simulink model "leg_contral_from_joy"  (R2024a)
settings: Solver=FixedStepDiscrete  StartTime=0.0  StopTime=inf  FixedStep=0.01  RelTol=1e-3  EnableMultiTasking=on
InitFcn:
  | run('robota_init.m')
values from neighbouring files (symbols this model uses):
  foot_step_x = single([0.647962241881123,0.669281948440417,0.689047458853030,0.707336632089232,0.724214871275340,0.739734081466605,0.753932398834638,0.766834545548556,0.778452679930586,0.788787625824203,0.797830378556315,0.805563797434742,0.811964406427908,0.817004235554845,0.820652645599333,0.822878088081130,0.823649760998204,0.822939128724922,0.820721281639968,0.816976117592065,0.811689333218330,0.804853218436 ...(+3308 chars)    [robota_init.m]
  foot_step_y = single([0.00431677655718721,0.0162618273816606,0.0344599539851875,0.0576998848000865,0.0849190036162384,0.115189239656799,0.147704049746776,0.181766425758056,0.216777863221598,0.252228229678260,0.287686473989677,0.322792120445942,0.357247494083859,0.390810626164481,0.423288791248474,0.454532629749211,0.484430812233581,0.512905204076631,0.539906491355785,0.565410231091200,0.589413291098898,0.611930 ...(+3410 chars)    [robota_init.m]
  height_plane = 0.025    [robota_init.m]
undefined symbols (not defined in the file or in its folder): axes, axes_SL_Info, buttons, buttons_SL_Info, foot_z, header, lb_alfa, lb_beta, lb_gamma, lf_alfa, lf_beta, lf_gamma, plane_x, plane_y, rb_alfa, rb_beta, rb_gamma, rf_alfa, rf_beta, rf_gamma, x, X, y, Y, z, Z
libraries: sm_lib x84, nesl_utility x21, hdlsllib x20, ros2lib x10, instrumentseriallib x2
(part 1 of 3)
settings Model: SimulationMode=external  Creator=The MathWorks, Inc.  LastModifiedBy=yang
settings SolverCC: AlgebraicLoopSolver=TrustRegion  PositivePriorityOrder=on
settings DataIOCC: LimitDataPoints=on  SaveFormat=Array  ReturnWorkspaceOutputs=off
settings OptimizationCC: ZeroExternalMemoryAtStartup=off  ZeroInternalMemoryAtStartup=off  LifeSpan=1  MaxStackSize=64
settings DebuggingCC: SolverPrmCheckMsg=warning  UnconnectedInputMsg=warning  UnconnectedOutputMsg=warning  UnconnectedLineMsg=warning  SFUnexpectedBacktrackingDiag=warning  SFNoUnconditionalDefaultTransitionDiag=warning  SFExecutionAtInitializationDiag=none  ArithmeticOperatorsInVariantConditions=warning
settings HardwareCC: ProdBitPerLong=64  ProdHWDeviceType=AMD->x86-64 (Linux 64)  TargetHWDeviceType=Generic->Unspecified (assume 32-bit Generic)
settings ModelReferenceCC: EnableRefExpFcnMdlSchedulingChecks=on  ModelReferenceNumInstancesAllowed=Single  PropagateSignalLabelsOutOfModel=off
settings SFSimCC: SimUseLocalCustomCode=off  SimTargetLang=C++
settings RTWCC: Description=Embedded Coder  SystemTargetFile=ert.tlc  HardwareBoard=Robot Operating System 2 (ROS 2)  TLCOptions="-aInlineSetEventsForThisBaseRateFcn=TLC_FALSE -aSuppressMultiTaskScheduler=TLC_FALSE   -aRateBasedStepFcn=0"  TemplateMakefile=ert_default_tmf  RTWUseLocalCustomCode=off  Toolchain=Colcon Tools  TargetLang=C++  GPUComputeCapability=3.5
settings CodeAppCC: StateflowObjectComments=on
settings ERTTargetCC: MultiwordLength=2048  ERTCustomFileBanners=off  CodeInterfacePackaging=C++ class  SupportContinuousTime=on  SupportNonInlinedSFcns=on  RemoveResetFunc=off  SupportVariableSizeSignals=on  ModelStepFunctionPrototypeControlCompliant=off  RootIOFormat=Structure reference  ConvertIfToSwitch=off  SuppressUnreachableDefaultCases=off
settings ConfigComp: CovMetricSettings=dw  CovSaveCumulativeToWorkspaceVar=on  CovSaveSingleToWorkspaceVar=on  CovExternalEMLEnable=off  CovSFcnEnable=off

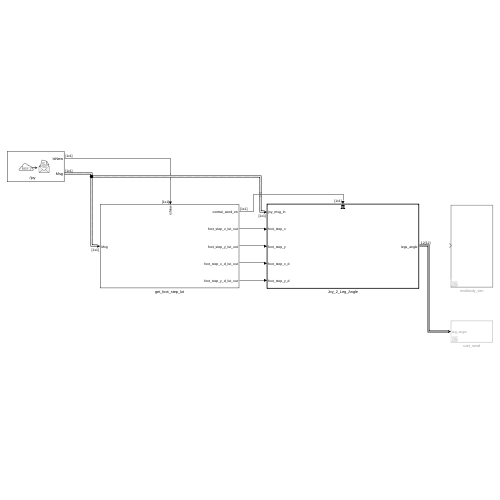
[thumbnail: Simulink's stored preview of the top-level diagram]
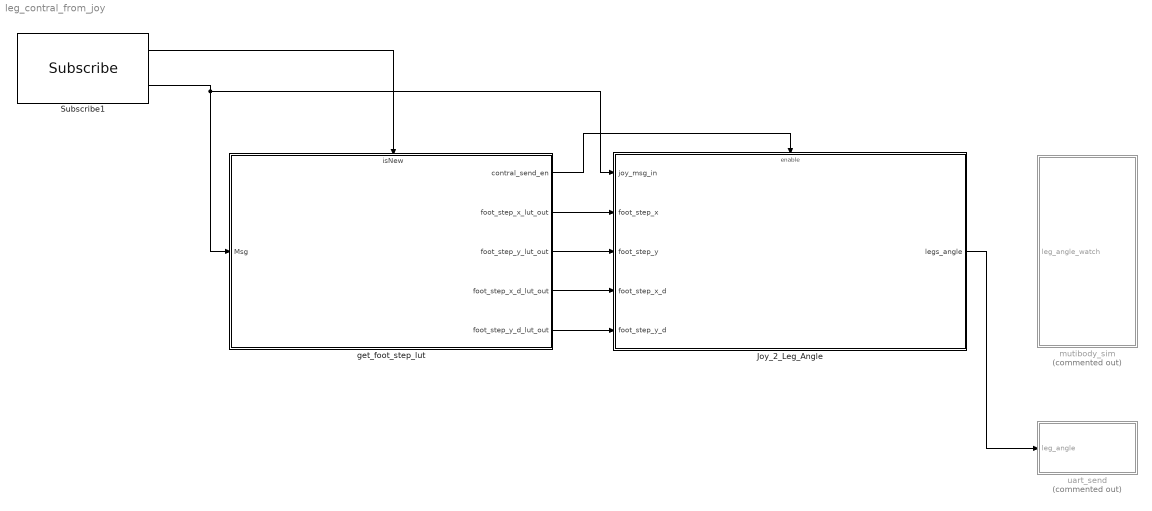
== system leg_contral_from_joy ==
  Joy_2_Leg_Angle : Subsystem
  Subscribe1 : ros2lib/Subscribe  topicSource=Select from ROS network  topic=/joy  messageType=sensor_msgs/Joy  sampleTime=0.01  QOSHistory=Keep last  QOSDepth=1  QOSReliability=Reliable  QOSDurability=Volatile  QOSDeadline=Inf  QOSLifespan=Inf  QOSLiveliness=Automatic  QOSLeaseDuration=Inf  QOSAvoidROSNamespaceConventions=off
  get_foot_step_lut : Subsystem
      settings: PortSchema="{\"entries\":[{\"content\":{\"sides\":[{\"content\":{\"connectorIds\":[\"In1\"]},\"type\":\"ConnectorPlacement.EquallySpacedRectSide\",\"uuid\":\"62496544-86df-4f58-acc1-b6358197f44c\"},{\"content\":{\"connectorIds\":[\"Out1\",\"Out2\",\"Out3\",\"Out4\",\"Out5\"],\"side\":\"RIGHT\"},\"type\":\"ConnectorPlacement.EquallySpacedRectSide\",\"uuid\":\"00f5c7b2-a8b0-46a5-a80f-764e0da961ac\"},{\"content\":{\"connectorIds\":[\"In2\"],\"side\":\"TOP\"},\"type\":\"ConnectorPlacement.EquallySpacedRectSide\",\"uuid\":\"1933786d-7f7d-47a2-bd92-b828693c7f9d\"}]},\"type\":\"ConnectorPlacement.EquallySpacedConnector\",\"uuid\":\"7dc846c5-42fe-4877-a1f3-97792b9a7f59\"}],\"packageUris\":[\"http://schema.mathworks.com/mf0/Connector/R2020b\"],\"version\":\"1.0\"}"
  mutibody_sim : Subsystem  Commented=on  TreatAsAtomicUnit=on
  uart_send : Subsystem  Commented=on
  wires:
  Subscribe1/2 -> Joy_2_Leg_Angle/1(joy_msg_in), get_foot_step_lut/1(Msg)
  Subscribe1/1 -> get_foot_step_lut/2(isNew)
  get_foot_step_lut/1(contral_send_en) -> Joy_2_Leg_Angle/Enable
  get_foot_step_lut/2(foot_step_x_lut_out) -> Joy_2_Leg_Angle/2(foot_step_x)
  get_foot_step_lut/3(foot_step_y_lut_out) -> Joy_2_Leg_Angle/3(foot_step_y)
  get_foot_step_lut/4(foot_step_x_d_lut_out) -> Joy_2_Leg_Angle/4(foot_step_x_d)
  get_foot_step_lut/5(foot_step_y_d_lut_out) -> Joy_2_Leg_Angle/5(foot_step_y_d)
  Joy_2_Leg_Angle/1(legs_angle) -> uart_send/1(leg_angle)

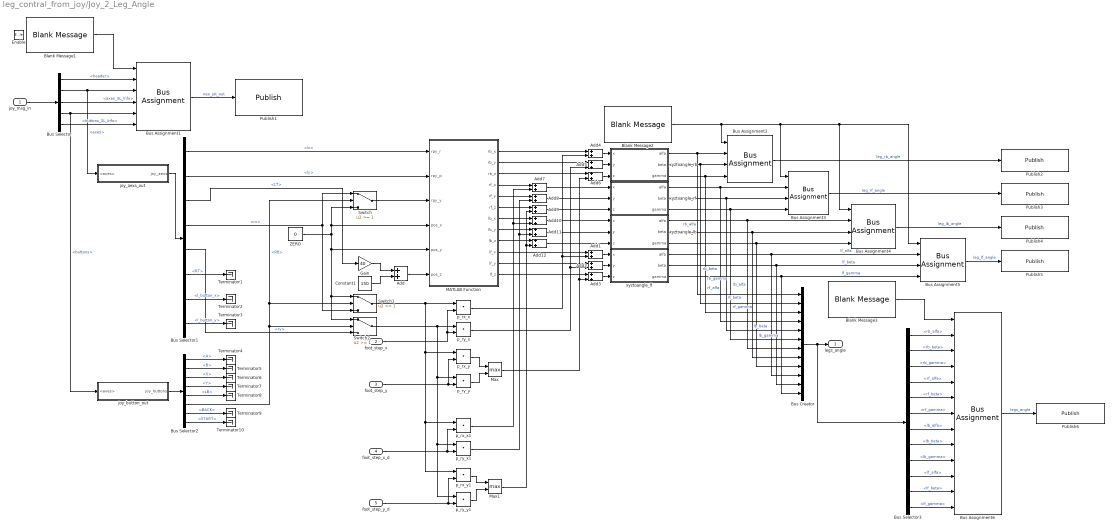
== system leg_contral_from_joy/Joy_2_Leg_Angle ==
  joy_msg_in : Inport
  foot_step_x : Inport  Port=2
  foot_step_y : Inport  Port=3
  foot_step_x_d : Inport  Port=4
  foot_step_y_d : Inport  Port=5
  Enable : EnablePort
  Add{,1..12} (13 alike) : Sum
  Blank Message1 : ros2lib/Blank Message  messageClass=Message  entityType=sensor_msgs/Joy  messageType=sensor_msgs/Joy  SampleTime=0.01
  Blank Message2 : ros2lib/Blank Message  messageClass=Message  entityType=geometry_msgs/Vector3  messageType=geometry_msgs/Vector3  SampleTime=0.01
  Blank Message3 : ros2lib/Blank Message  messageClass=Message  entityType=robota_leg_pos/LegPos  messageType=robota_leg_pos/LegPos  SampleTime=0.01
  Bus Assignment1 : BusAssignment  AssignedSignals=header,axes,axes_SL_Info,buttons,buttons_SL_Info
  Bus Assignment{2..5} (4 alike) : BusAssignment  AssignedSignals=x,y,z
  Bus Assignment6 : BusAssignment  AssignedSignals=rb_alfa,rb_beta,rb_gamma,rf_alfa,rf_beta,rf_gamma,lb_alfa,lb_beta,lb_gamma,lf_alfa,lf_beta,lf_gamma
  Bus Creator : BusCreator  Inputs=12
  Bus Selector : BusSelector  DialogController=Simulink.DDGSource_BusSelector  OutputSignals=header,axes,axes_SL_Info,buttons,buttons_SL_Info
  Bus Selector1 : BusSelector  OutputSignals=lx,ly,LT,rx,ry,RT,l_button_x,l_button_y
  Bus Selector2 : BusSelector  OutputSignals=A,B,X,Y,LB,RB,BACK,START
  Bus Selector3 : BusSelector  OutputSignals=rb_alfa,rb_beta,rb_gamma,rf_alfa,rf_beta,rf_gamma,lb_alfa,lb_beta,lb_gamma,lf_alfa,lf_beta,lf_gamma
  Constant1 : Constant  Value=150  SampleTime=0.01
  Gain : Gain  Gain=40
  MATLAB Function : MATLAB Function  TreatAsAtomicUnit=on
  Max : MinMax  Function=max  Inputs=2
  Max1 : MinMax  Function=max  Inputs=2
  Publish1 : ros2lib/Publish  topicSource=Specify your own  topic=/joy_neo  messageType=sensor_msgs/Joy  QOSHistory=Keep last  QOSDepth=10  QOSReliability=Reliable  QOSDurability=Volatile  QOSDeadline=Inf  QOSLifespan=Inf  QOSLiveliness=Automatic  QOSLeaseDuration=Inf  QOSAvoidROSNamespaceConventions=off
  Publish2 : ros2lib/Publish  topicSource=Specify your own  topic=/leg_rb_angle  messageType=geometry_msgs/Vector3  QOSHistory=Keep last  QOSDepth=10  QOSReliability=Reliable  QOSDurability=Volatile  QOSDeadline=Inf  QOSLifespan=Inf  QOSLiveliness=Automatic  QOSLeaseDuration=Inf  QOSAvoidROSNamespaceConventions=off
  Publish3 : ros2lib/Publish  topicSource=Specify your own  topic=/leg_rf_angle  messageType=geometry_msgs/Vector3  QOSHistory=Keep last  QOSDepth=10  QOSReliability=Reliable  QOSDurability=Volatile  QOSDeadline=Inf  QOSLifespan=Inf  QOSLiveliness=Automatic  QOSLeaseDuration=Inf  QOSAvoidROSNamespaceConventions=off
  Publish4 : ros2lib/Publish  topicSource=Specify your own  topic=/leg_lb_angle  messageType=geometry_msgs/Vector3  QOSHistory=Keep last  QOSDepth=10  QOSReliability=Reliable  QOSDurability=Volatile  QOSDeadline=Inf  QOSLifespan=Inf  QOSLiveliness=Automatic  QOSLeaseDuration=Inf  QOSAvoidROSNamespaceConventions=off
  Publish5 : ros2lib/Publish  topicSource=Specify your own  topic=/leg_lf_angle  messageType=geometry_msgs/Vector3  QOSHistory=Keep last  QOSDepth=10  QOSReliability=Reliable  QOSDurability=Volatile  QOSDeadline=Inf  QOSLifespan=Inf  QOSLiveliness=Automatic  QOSLeaseDuration=Inf  QOSAvoidROSNamespaceConventions=off
  Publish6 : ros2lib/Publish  topicSource=Specify your own  topic=/legs_angle  messageType=robota_leg_pos/LegPos  QOSHistory=Keep last  QOSDepth=10  QOSReliability=Reliable  QOSDurability=Volatile  QOSDeadline=Inf  QOSLifespan=Inf  QOSLiveliness=Automatic  QOSLeaseDuration=Inf  QOSAvoidROSNamespaceConventions=off
  Switch : Switch  Threshold=1  SaturateOnIntegerOverflow=off  InputSameDT=off
  Switch1 : Switch  Threshold=1  SaturateOnIntegerOverflow=off  InputSameDT=off
  Switch2 : Switch  Threshold=1  SaturateOnIntegerOverflow=off  InputSameDT=off
  Terminator{1..10} (10 alike) : Terminator
  ZERO : Constant  Value=0  SampleTime=0.01
  joy_aexs_out : Subsystem
  joy_button_out : Subsystem
  p_rx_x : DotProduct  OutDataTypeStr=single
  p_rx_x1 : DotProduct  OutDataTypeStr=Inherit: Inherit via internal rule
  p_rx_y : DotProduct  OutDataTypeStr=Inherit: Inherit via internal rule
  p_rx_y1 : DotProduct  OutDataTypeStr=Inherit: Inherit via internal rule
  p_ry_x : DotProduct  OutDataTypeStr=Inherit: Inherit via internal rule
  p_ry_x1 : DotProduct  OutDataTypeStr=Inherit: Inherit via internal rule
  p_ry_y : DotProduct  OutDataTypeStr=Inherit: Inherit via internal rule
  p_ry_y1 : DotProduct  OutDataTypeStr=Inherit: Inherit via internal rule
  xyztoangle_lb : MATLAB Function  TreatAsAtomicUnit=on
  xyztoangle_lf : MATLAB Function  TreatAsAtomicUnit=on
  xyztoangle_rb : MATLAB Function  TreatAsAtomicUnit=on
  xyztoangle_rf : MATLAB Function  TreatAsAtomicUnit=on
  legs_angle : Outport
  wires:
  joy_msg_in/1 -> Bus Selector/1
  Bus Selector/2 -> Bus Assignment1/3, joy_aexs_out/1(<axes>)  "<axes>"
  Blank Message1/1 -> Bus Assignment1/1
  Bus Assignment1/1 -> Publish1/1  "neo_jot_out"
  Bus Selector/4 -> joy_button_out/1(<axes>), Bus Assignment1/5  "<buttons>"
  Bus Selector/1 -> Bus Assignment1/2  "<header>"
  Bus Selector/3 -> Bus Assignment1/4  "<axes_SL_Info>"
  Bus Selector/5 -> Bus Assignment1/6  "<buttons_SL_Info>"
  MATLAB Function/1(rb_x) -> Add4/1
  MATLAB Function/2(rb_y) -> Add5/1
  MATLAB Function/3(rb_z) -> Add6/1
  MATLAB Function/4(rf_x) -> Add7/1
  MATLAB Function/5(rf_y) -> Add8/1
  MATLAB Function/6(rf_z) -> Add9/1
  MATLAB Function/7(lb_x) -> Add10/1
  MATLAB Function/8(lb_y) -> Add11/1
  MATLAB Function/9(lb_z) -> Add12/1
  MATLAB Function/10(lf_x) -> Add1/1
  MATLAB Function/11(lf_y) -> Add2/1
  MATLAB Function/12(lf_z) -> Add3/1
  joy_aexs_out/1(joy_aexs) -> Bus Selector1/1
  Bus Selector1/1 -> MATLAB Function/1(rpy_r)  "<lx>"
  Bus Selector1/2 -> MATLAB Function/2(rpy_p)  "<ly>"
  Bus Selector1/3 -> Gain/1  "<LT>"
  Bus Selector1/6 -> Terminator1/1  "<RT>"
  Bus Selector1/8 -> Terminator3/1  "<l_button_y>"
  ZERO/1 -> MATLAB Function/5(pos_y), Switch2/1, Switch1/1, MATLAB Function/4(pos_x), Switch/3
  Add/1 -> MATLAB Function/6(pos_z)
  Blank Message2/1 -> Bus Assignment5/1, Bus Assignment4/1, Bus Assignment3/1, Bus Assignment2/1
  xyztoangle_rb/1(alfa) -> Bus Creator/1, Bus Assignment2/2  "rb_alfa"
  xyztoangle_rb/2(beta) -> Bus Creator/2, Bus Assignment2/3  "rb_beta"
  xyztoangle_rb/3(gamma) -> Bus Creator/3, Bus Assignment2/4  "rb_gamma"
  Bus Assignment2/1 -> Publish2/1  "leg_rb_angle"
  Bus Assignment3/1 -> Publish3/1  "leg_rf_angle"
  xyztoangle_rf/1(alfa) -> Bus Creator/4, Bus Assignment3/2  "rf_alfa"
  xyztoangle_rf/2(beta) -> Bus Creator/5, Bus Assignment3/3  "rf_beta"
  xyztoangle_rf/3(gamma) -> Bus Creator/6, Bus Assignment3/4  "rf_gamma"
  Bus Assignment5/1 -> Publish5/1  "leg_lf_angle"
  Bus Assignment4/1 -> Publish4/1  "leg_lb_angle"
  xyztoangle_lb/1(alfa) -> Bus Creator/7, Bus Assignment4/2  "lb_alfa"
  xyztoangle_lb/2(beta) -> Bus Creator/8, Bus Assignment4/3  "lb_beta"
  xyztoangle_lb/3(gamma) -> Bus Creator/9, Bus Assignment4/4  "lb_gamma"
  xyztoangle_lf/1(alfa) -> Bus Creator/10, Bus Assignment5/2  "lf_alfa"
  xyztoangle_lf/2(beta) -> Bus Creator/11, Bus Assignment5/3  "lf_beta"
  xyztoangle_lf/3(gamma) -> Bus Creator/12, Bus Assignment5/4  "lf_gamma"
  joy_button_out/1(joy_buttons) -> Bus Selector2/1
  Bus Selector2/1 -> Terminator4/1  "<A>"
  Bus Selector2/2 -> Terminator5/1  "<B>"
  Bus Selector2/3 -> Terminator6/1  "<X>"
  Bus Selector2/4 -> Terminator7/1  "<Y>"
  Bus Selector2/5 -> Terminator8/1  "<LB>"
  Bus Selector2/6 -> Switch1/2, Switch/2, Switch2/2  "<RB>"
  Bus Selector2/7 -> Terminator9/1  "<BACK>"
  Bus Selector2/8 -> Terminator10/1  "<START>"
  Switch/1 -> MATLAB Function/3(rpy_y)
  Constant1/1 -> Add/2
  Gain/1 -> Add/1
  Add1/1 -> xyztoangle_lf/1(x)
  Add2/1 -> xyztoangle_lf/2(y)
  Add3/1 -> xyztoangle_lf/3(z)
  foot_step_y/1 -> p_rx_y/2, p_ry_y/2
  p_rx_y/1 -> Max/1
  foot_step_x/1 -> p_rx_x/2, p_ry_x/2
  p_rx_x/1 -> Add4/2, Add1/2
  Max/1 -> Add6/2, Add3/2
  p_ry_y/1 -> Max/2
  p_ry_x/1 -> Add5/2, Add2/2
  Add4/1 -> xyztoangle_rb/1(x)
  Add5/1 -> xyztoangle_rb/2(y)
  Add6/1 -> xyztoangle_rb/3(z)
  foot_step_x_d/1 -> p_rx_x1/2, p_ry_x1/2
  foot_step_y_d/1 -> p_rx_y1/2, p_ry_y1/2
  Switch2/1 -> p_ry_x/1, p_ry_x1/1, p_ry_y1/1, p_ry_y/1
  Switch1/1 -> p_rx_y/1, p_rx_y1/1, p_rx_x1/1, p_rx_x/1
  p_rx_y1/1 -> Max1/1
  p_ry_y1/1 -> Max1/2
  Add7/1 -> xyztoangle_rf/1(x)
  Add8/1 -> xyztoangle_rf/2(y)
  Add9/1 -> xyztoangle_rf/3(z)
  Add10/1 -> xyztoangle_lb/1(x)
  Add11/1 -> xyztoangle_lb/2(y)
  Add12/1 -> xyztoangle_lb/3(z)
  p_rx_x1/1 -> Add10/2, Add7/2
  p_ry_x1/1 -> Add8/2, Add11/2
  Max1/1 -> Add9/2, Add12/2
  Bus Selector1/7 -> Terminator2/1  "<l_button_x>"
  Bus Selector1/4 -> Switch/1, Switch1/3  "<rx>"
  Bus Selector1/5 -> Switch2/3  "<ry>"
  Bus Creator/1 -> Bus Selector3/1, legs_angle/1
  Blank Message3/1 -> Bus Assignment6/1
  Bus Assignment6/1 -> Publish6/1  "legs_angle"
  Bus Selector3/1 -> Bus Assignment6/2  "<rb_alfa>"
  Bus Selector3/2 -> Bus Assignment6/3  "<rb_beta>"
  Bus Selector3/3 -> Bus Assignment6/4  "<rb_gamma>"
  Bus Selector3/4 -> Bus Assignment6/5  "<rf_alfa>"
  Bus Selector3/5 -> Bus Assignment6/6  "<rf_beta>"
  Bus Selector3/6 -> Bus Assignment6/7  "<rf_gamma>"
  Bus Selector3/7 -> Bus Assignment6/8  "<lb_alfa>"
  Bus Selector3/8 -> Bus Assignment6/9  "<lb_beta>"
  Bus Selector3/9 -> Bus Assignment6/10  "<lb_gamma>"
  Bus Selector3/10 -> Bus Assignment6/11  "<lf_alfa>"
  Bus Selector3/11 -> Bus Assignment6/12  "<lf_beta>"
  Bus Selector3/12 -> Bus Assignment6/13  "<lf_gamma>"

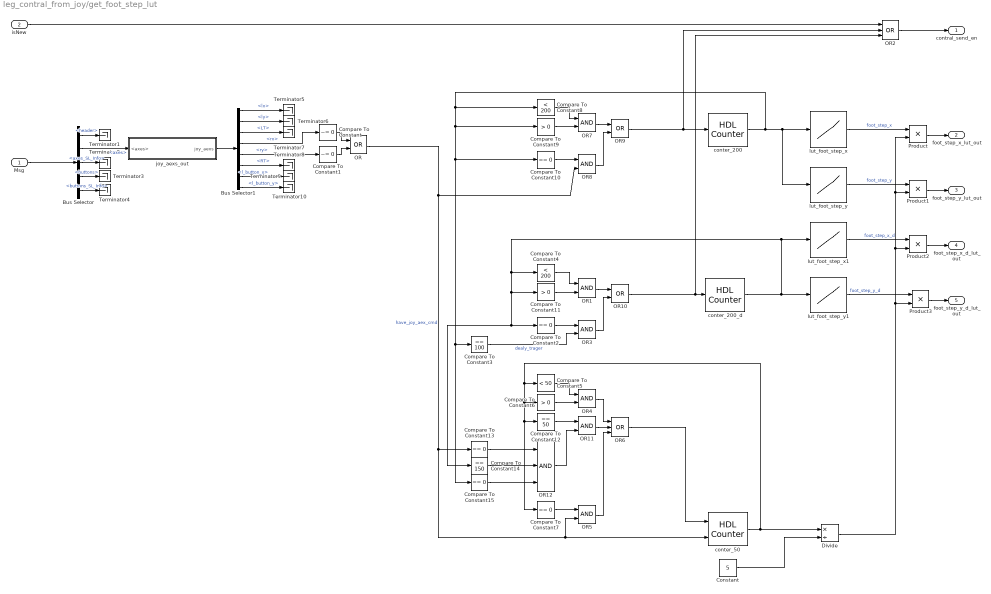
== system leg_contral_from_joy/get_foot_step_lut ==
  Msg : Inport
  isNew : Inport  Port=2
  Bus Selector : BusSelector  DialogController=Simulink.DDGSource_BusSelector  OutputSignals=header,axes,axes_SL_Info,buttons,buttons_SL_Info
  Bus Selector1 : BusSelector  OutputSignals=lx,ly,LT,rx,ry,RT,l_button_x,l_button_y
  Compare To Constant : hdlsllib/Logic and Bit Operations/Compare To Constant  relop=~=  const=0  OutDataTypeStr=boolean
  Compare To Constant1 : hdlsllib/Logic and Bit Operations/Compare To Constant  relop=~=  const=0  OutDataTypeStr=boolean
  Compare To Constant{2,7,10,13,15} (5 alike) : hdlsllib/Logic and Bit Operations/Compare To Constant  relop===  const=0  OutDataTypeStr=boolean
  Compare To Constant11 : hdlsllib/Logic and Bit Operations/Compare To Constant  relop=>  const=0  OutDataTypeStr=boolean
  Compare To Constant12 : hdlsllib/Logic and Bit Operations/Compare To Constant  relop===  const=50  OutDataTypeStr=boolean
  Compare To Constant14 : hdlsllib/Logic and Bit Operations/Compare To Constant  relop===  const=150  OutDataTypeStr=boolean
  Compare To Constant3 : hdlsllib/Logic and Bit Operations/Compare To Constant  relop===  const=100  OutDataTypeStr=boolean
  Compare To Constant4 : hdlsllib/Logic and Bit Operations/Compare To Constant  relop=<  const=200  OutDataTypeStr=boolean
  Compare To Constant5 : hdlsllib/Logic and Bit Operations/Compare To Constant  relop=<  const=50  OutDataTypeStr=boolean
  Compare To Constant6 : hdlsllib/Logic and Bit Operations/Compare To Constant  relop=>  const=0  OutDataTypeStr=boolean
  Compare To Constant8 : hdlsllib/Logic and Bit Operations/Compare To Constant  relop=<  const=200  OutDataTypeStr=boolean
  Compare To Constant9 : hdlsllib/Logic and Bit Operations/Compare To Constant  relop=>  const=0  OutDataTypeStr=boolean
  Constant : Constant  Value=5  SampleTime=0.01
  Divide : Product  Inputs=*/
  OR : Logic  Operator=OR  AllPortsSameDT=off  OutDataTypeStr=boolean
  OR{1,3..5,7..8,11} (7 alike) : Logic  AllPortsSameDT=off  OutDataTypeStr=boolean
  OR10 : Logic  Operator=OR  AllPortsSameDT=off  OutDataTypeStr=boolean
  OR12 : Logic  Inputs=3  AllPortsSameDT=off  OutDataTypeStr=boolean
  OR2 : Logic  Operator=OR  Inputs=3  AllPortsSameDT=off  OutDataTypeStr=boolean
  OR6 : Logic  Operator=OR  Inputs=3  AllPortsSameDT=off  OutDataTypeStr=boolean
  OR9 : Logic  Operator=OR  AllPortsSameDT=off  OutDataTypeStr=boolean
  Product{,1..3} (4 alike) : Product  OutDataTypeStr=single
  Terminator{1..10} (10 alike) : Terminator
  conter_200 : hdlsllib/Sources/HDL Counter  CountType=Count limited  CountInit=0  CountStep=1  CountMax=199  CountFromType=Initial value  CountFrom=0  CountResetPort=off  CountLoadPort=off  CountEnbPort=on  CountDirPort=off  CountHitOutputPort=off  CountDataType=Unsigned  CountWordLen=8  CountFracLen=0  CountSampTime=1
  conter_200_d : hdlsllib/Sources/HDL Counter  CountType=Count limited  CountInit=0  CountStep=1  CountMax=199  CountFromType=Initial value  CountFrom=0  CountResetPort=off  CountLoadPort=off  CountEnbPort=on  CountDirPort=off  CountHitOutputPort=off  CountDataType=Unsigned  CountWordLen=8  CountFracLen=0  CountSampTime=1
  conter_50 : hdlsllib/Sources/HDL Counter  CountType=Modulo  CountInit=0  CountStep=1  CountMax=50  CountFromType=Initial value  CountFrom=0  CountResetPort=off  CountLoadPort=off  CountEnbPort=on  CountDirPort=on  CountHitOutputPort=off  CountDataType=Unsigned  CountWordLen=8  CountFracLen=0  CountSampTime=1
  joy_aexs_out : Subsystem
  lut_foot_step_x : Lookup_n-D  NumberOfTableDimensions=1  BreakpointsForDimension1=[0:199]  BreakpointsForDimension1DataTypeStr=single  Table=foot_step_x  TableDataTypeStr=single  IntermediateResultsDataTypeStr=single  ExtrapMethod=Clip  InternalRulePriority=Speed  OutDataTypeStr=single  RndMeth=Simplest  FractionDataTypeStr=single
  lut_foot_step_x1 : Lookup_n-D  NumberOfTableDimensions=1  BreakpointsForDimension1=[0:199]  BreakpointsForDimension1DataTypeStr=single  Table=foot_step_x  TableDataTypeStr=single  IntermediateResultsDataTypeStr=single  ExtrapMethod=Clip  InternalRulePriority=Speed  OutDataTypeStr=single  RndMeth=Simplest  FractionDataTypeStr=single
  lut_foot_step_y : Lookup_n-D  NumberOfTableDimensions=1  BreakpointsForDimension1=[0:199]  BreakpointsForDimension1DataTypeStr=single  Table=foot_step_y  TableDataTypeStr=single  IntermediateResultsDataTypeStr=single  ExtrapMethod=Clip  InternalRulePriority=Speed  OutDataTypeStr=single  RndMeth=Simplest  FractionDataTypeStr=single
  lut_foot_step_y1 : Lookup_n-D  NumberOfTableDimensions=1  BreakpointsForDimension1=[0:199]  BreakpointsForDimension1DataTypeStr=single  Table=foot_step_y  TableDataTypeStr=single  IntermediateResultsDataTypeStr=single  ExtrapMethod=Clip  InternalRulePriority=Speed  OutDataTypeStr=single  RndMeth=Simplest  FractionDataTypeStr=single
  contral_send_en : Outport
  foot_step_x_lut_out : Outport  Port=2
  foot_step_y_lut_out : Outport  Port=3
  foot_step_x_d_lut_out : Outport  Port=4
  foot_step_y_d_lut_out : Outport  Port=5
  wires:
  Compare To Constant13/1 -> OR12/1
  OR8/1 -> OR9/2
  Compare To Constant5/1 -> OR4/1
  Bus Selector1/1 -> Terminator5/1  "<lx>"
  lut_foot_step_x1/1 -> Product2/1  "foot_step_x_d"
  Bus Selector1/6 -> Terminator8/1  "<RT>"
  Compare To Constant9/1 -> OR7/2
  Compare To Constant10/1 -> OR8/1
  Bus Selector1/2 -> Terminator6/1  "<ly>"
  Compare To Constant7/1 -> OR5/1
  Bus Selector1/3 -> Terminator7/1  "<LT>"
  Compare To Constant2/1 -> OR3/1
  Bus Selector/4 -> Terminator3/1  "<buttons>"
  Msg/1 -> Bus Selector/1
  lut_foot_step_x/1 -> Product/1  "foot_step_x"
  OR6/1 -> conter_50/1
  Constant/1 -> Divide/2
  OR11/1 -> OR6/2
  Bus Selector/2 -> joy_aexs_out/1(<axes>)  "<axes>"
  Bus Selector/1 -> Terminator1/1  "<header>"
  Product/1 -> foot_step_x_lut_out/1
  OR2/1 -> contral_send_en/1
  Bus Selector1/4 -> Compare To Constant/1  "<rx>"
  Compare To Constant15/1 -> OR12/3
  Compare To Constant11/1 -> OR1/2
  OR/1 -> OR5/2, conter_50/2, Compare To Constant13/1, OR8/2  "have_joy_aex_cmd"
  Compare To Constant/1 -> OR/1
  conter_200_d/1 -> Compare To Constant2/1, Compare To Constant14/1, Compare To Constant11/1, Compare To Constant4/1, lut_foot_step_x1/1, lut_foot_step_y1/1
  Divide/1 -> Product3/2, Product2/2, Product1/2, Product/2
  conter_200/1 -> Compare To Constant15/1, Compare To Constant3/1, Compare To Constant10/1, Compare To Constant9/1, Compare To Constant8/1, lut_foot_step_y/1, lut_foot_step_x/1
  Compare To Constant3/1 -> OR3/2  "dealy_trager"
  OR3/1 -> OR10/2
  Compare To Constant12/1 -> OR11/1
  isNew/1 -> OR2/1
  lut_foot_step_y1/1 -> Product3/1  "foot_step_y_d"
  Product2/1 -> foot_step_x_d_lut_out/1
  Compare To Constant1/1 -> OR/2
  Bus Selector/3 -> Terminator2/1  "<axes_SL_Info>"
  OR1/1 -> OR10/1
  Product3/1 -> foot_step_y_d_lut_out/1
  Bus Selector1/5 -> Compare To Constant1/1  "<ry>"
  conter_50/1 -> Divide/1, Compare To Constant7/1, Compare To Constant12/1, Compare To Constant6/1, Compare To Constant5/1
  OR5/1 -> OR6/3
  OR10/1 -> OR2/3, conter_200_d/1
  OR12/1 -> OR11/2
  OR4/1 -> OR6/1
  joy_aexs_out/1(joy_aexs) -> Bus Selector1/1
  Compare To Constant6/1 -> OR4/2
  lut_foot_step_y/1 -> Product1/1  "foot_step_y"
  Bus Selector1/7 -> Terminator9/1  "<l_button_x>"
  OR9/1 -> conter_200/1, OR2/2
  Compare To Constant8/1 -> OR7/1
  OR7/1 -> OR9/1
  Bus Selector/5 -> Terminator4/1  "<buttons_SL_Info>"
  Compare To Constant4/1 -> OR1/1
  Product1/1 -> foot_step_y_lut_out/1
  Compare To Constant14/1 -> OR12/2
  Bus Selector1/8 -> Terminator10/1  "<l_button_y>"

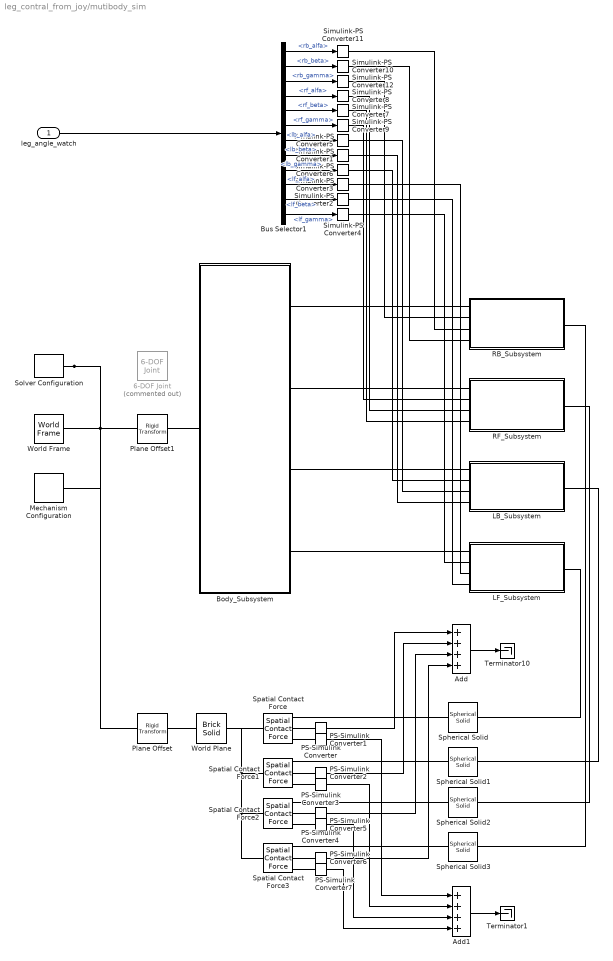
== system leg_contral_from_joy/mutibody_sim ==
  leg_angle_watch : Inport
  6-DOF Joint : sm_lib/Joints/6-DOF Joint  Commented=on  JointMode=Normal  CompositeWrenchDir=FollowerOnBase  CompositeWrenchFrame=BaseFrame  SenseConstraintForce=off  SenseConstraintTorque=off  SenseTotalForce=off  SenseTotalTorque=off  PxPositionTargetSpecify=off  PxPositionTargetPriority=High  PxPositionTargetValue=0  PxPositionTargetValueUnits=m  PxVelocityTargetSpecify=off  PxVelocityTargetPriority=High  PxVelocityTargetValue=0  PxVelocityTargetValueUnits=m/s  PxEquilibriumPosition=0  PxEquilibriumPositionUnits=m  PxSpringStiffness=0  PxSpringStiffnessUnits=N/m  PxDampingCoefficient=0  PxDampingCoefficientUnits=N/(m/s)  PxLowerLimitSpecify=off  PxLowerLimitBound=-1  PxLowerLimitBoundUnits=m  PxLowerLimitStiffness=1e6  PxLowerLimitStiffnessUnits=N/m  PxLowerLimitDamping=1e3  PxLowerLimitDampingUnits=N/(m/s)  PxLowerLimitTransitionRegionWidth=1e-4  PxLowerLimitTransitionRegionWidthUnits=m  PxUpperLimitSpecify=off  PxUpperLimitBound=1  PxUpperLimitBoundUnits=m  PxUpperLimitStiffness=1e6  PxUpperLimitStiffnessUnits=N/m  PxUpperLimitDamping=1e3  PxUpperLimitDampingUnits=N/(m/s)  PxUpperLimitTransitionRegionWidth=1e-4  PxUpperLimitTransitionRegionWidthUnits=m  PxTorqueActuationMode=NoTorque  PxMotionActuationMode=ComputedMotion  PxSensePosition=off  PxSenseVelocity=off  PxSenseAcceleration=off  PxSenseTorqueForce=off  PxSenseLowerLimitTorqueForce=off  PxSenseUpperLimitTorqueForce=off  PyPositionTargetSpecify=off  PyPositionTargetPriority=High  PyPositionTargetValue=0  PyPositionTargetValueUnits=m  PyVelocityTargetSpecify=off  PyVelocityTargetPriority=High  PyVelocityTargetValue=0  PyVelocityTargetValueUnits=m/s  PyEquilibriumPosition=0  PyEquilibriumPositionUnits=m  PySpringStiffness=0  PySpringStiffnessUnits=N/m  PyDampingCoefficient=0  PyDampingCoefficientUnits=N/(m/s)  PyLowerLimitSpecify=off  PyLowerLimitBound=-1  PyLowerLimitBoundUnits=m  PyLowerLimitStiffness=1e6  PyLowerLimitStiffnessUnits=N/m  PyLowerLimitDamping=1e3  PyLowerLimitDampingUnits=N/(m/s)  PyLowerLimitTransitionRegionWidth=1e-4  PyLowerLimitTransitionRegionWidthUnits=m  PyUpperLimitSpecify=off  PyUpperLimitBound=1  PyUpperLimitBoundUnits=m  PyUpperLimitStiffness=1e6  PyUpperLimitStiffnessUnits=N/m  PyUpperLimitDamping=1e3  PyUpperLimitDampingUnits=N/(m/s)  PyUpperLimitTransitionRegionWidth=1e-4  PyUpperLimitTransitionRegionWidthUnits=m  PyTorqueActuationMode=NoTorque  PyMotionActuationMode=ComputedMotion  PySensePosition=off  PySenseVelocity=off  PySenseAcceleration=off  PySenseTorqueForce=off  PySenseLowerLimitTorqueForce=off  PySenseUpperLimitTorqueForce=off  PzPositionTargetSpecify=off  PzPositionTargetPriority=High  PzPositionTargetValue=0  PzPositionTargetValueUnits=m  PzVelocityTargetSpecify=off  PzVelocityTargetPriority=High  PzVelocityTargetValue=0  PzVelocityTargetValueUnits=m/s  PzEquilibriumPosition=0  PzEquilibriumPositionUnits=m  PzSpringStiffness=0  PzSpringStiffnessUnits=N/m  PzDampingCoefficient=0  PzDampingCoefficientUnits=N/(m/s)  PzLowerLimitSpecify=off  PzLowerLimitBound=-1  PzLowerLimitBoundUnits=m  PzLowerLimitStiffness=1e6  PzLowerLimitStiffnessUnits=N/m  PzLowerLimitDamping=1e3  PzLowerLimitDampingUnits=N/(m/s)  PzLowerLimitTransitionRegionWidth=1e-4  PzLowerLimitTransitionRegionWidthUnits=m  PzUpperLimitSpecify=off  PzUpperLimitBound=1  PzUpperLimitBoundUnits=m  PzUpperLimitStiffness=1e6  PzUpperLimitStiffnessUnits=N/m  PzUpperLimitDamping=1e3  PzUpperLimitDampingUnits=N/(m/s)  PzUpperLimitTransitionRegionWidth=1e-4  PzUpperLimitTransitionRegionWidthUnits=m  PzTorqueActuationMode=NoTorque  PzMotionActuationMode=ComputedMotion  PzSensePosition=off  PzSenseVelocity=off  PzSenseAcceleration=off  PzSenseTorqueForce=off  PzSenseLowerLimitTorqueForce=off  PzSenseUpperLimitTorqueForce=off  SphPositionTargetSpecify=off  SphPositionTargetPriority=High  SphPositionTargetRotationMethod=None  SphPositionTargetFollAlignAxisA=+X  SphPositionTargetBaseAlignAxisA=+Y  SphPositionTargetFollAlignAxisB=+Y  SphPositionTargetBaseAlignAxisB=+Z  SphPositionTargetRotationStandardAxis=+Z  SphPositionTargetRotationAngle=0.0  SphPositionTargetRotationAngleUnits=deg  SphPositionTargetRotationArbitraryAxis=[0 0 1]  SphPositionTargetRotationSequenceAxes=FollowerAxes  SphPositionTargetRotationSequence=XYX  SphPositionTargetRotationSequenceAngles=[0 0 0]  SphPositionTargetRotationSequenceAnglesUnits=deg  SphPositionTargetRotationMatrix=[1 0 0; 0 1 0; 0 0 1]  SphPositionTargetQuaternion=[1 0 0 0]  SphVelocityTargetSpecify=off  SphVelocityTargetPriority=High  SphVelocityTargetValue=[0 0 0]  SphVelocityTargetValueUnits=deg/s  SphVelocityTargetInFollowerFrame=on  SphEqPosRotationMethod=None  SphEqPosFollAlignAxisA=+X  SphEqPosBaseAlignAxisA=+Y  SphEqPosFollAlignAxisB=+Y  SphEqPosBaseAlignAxisB=+Z  SphEqPosRotationStandardAxis=+Z  SphEqPosRotationAngle=0.0  SphEqPosRotationAngleUnits=deg  SphEqPosRotationArbitraryAxis=[0 0 1]  SphEqPosRotationSequenceAxes=FollowerAxes  SphEqPosRotationSequence=XYX  SphEqPosRotationSequenceAngles=[0 0 0]  SphEqPosRotationSequenceAnglesUnits=deg  SphEqPosRotationMatrix=[1 0 0; 0 1 0; 0 0 1]  SphEqPosQuaternion=[1 0 0 0]  SphSpringStiffness=0  SphSpringStiffnessUnits=N*m/deg  SphDampingCoefficient=0  SphDampingCoefficientUnits=N*m/(deg/s)  SphLowerLimitSpecify=off  SphLowerLimitBound=15  SphLowerLimitBoundUnits=deg  SphLowerLimitStiffness=1e4  SphLowerLimitStiffnessUnits=N*m/deg  SphLowerLimitDamping=10  SphLowerLimitDampingUnits=N*m/(deg/s)  SphLowerLimitTransitionRegionWidth=0.1  SphLowerLimitTransitionRegionWidthUnits=deg  SphUpperLimitSpecify=off  SphUpperLimitBound=45  SphUpperLimitBoundUnits=deg  SphUpperLimitStiffness=1e4  SphUpperLimitStiffnessUnits=N*m/deg  SphUpperLimitDamping=10  SphUpperLimitDampingUnits=N*m/(deg/s)  SphUpperLimitTransitionRegionWidth=0.1  SphUpperLimitTransitionRegionWidthUnits=deg  SphTorqueActuationMode=NoTorque  SphActuateTorqueX=off  SphActuateTorqueY=off  SphActuateTorqueZ=off  SphActuateTorque=off  SphActuationFrame=BaseFrame  SphSensePosition=off  SphSenseVelocityX=off  SphSenseVelocityY=off  SphSenseVelocityZ=off  SphSenseVelocity=off  SphSenseAccelerationX=off  SphSenseAccelerationY=off  SphSenseAccelerationZ=off  SphSenseAcceleration=off  SphSenseLowerLimitTorqueMag=off  SphSenseUpperLimitTorqueMag=off  SphSensingFrame=BaseFrame
  Add : Sum  Inputs=4
  Add1 : Sum  Inputs=4
  Body_Subsystem : Subsystem
  Bus Selector1 : BusSelector  OutputSignals=rb_alfa,rb_beta,rb_gamma,rf_alfa,rf_beta,rf_gamma,lb_alfa,lb_beta,lb_gamma,lf_alfa,lf_beta,lf_gamma
  LB_Subsystem : Subsystem
  LF_Subsystem : Subsystem
  Mechanism Configuration : sm_lib/Utilities/Mechanism Configuration  UniformGravity=Constant  GravityVector=[0 0 -9.80665]  GravityVectorUnits=m/s^2  LinearizationDelta=0.001  JointModeTransitionNonlinearIterations=2
  PS-Simulink Converter{,1..7} (8 alike) : nesl_utility/PS-Simulink Converter  PhysicalDomain=network_engine_domain  SubClassName=ps_output  LeftPortType=input  RightPortType=output  PseudoPeriodic=off  Frequencies=[]  VectorFormat=1-D array  Unit=inherit  AffineConversion=off
  Plane Offset : sm_lib/Frames and Transforms/Rigid Transform  RotationMethod=None  FollAlignAxisA=+X  BaseAlignAxisA=+Y  FollAlignAxisB=+Y  BaseAlignAxisB=+Z  RotationStandardAxis=+Z  RotationAngle=0.0  RotationAngleUnits=deg  RotationArbitraryAxis=[0 0 1]  RotationSequenceAxes=FollowerAxes  RotationSequence=XYX  RotationSequenceAngles=[0 0 0]  RotationSequenceAnglesUnits=deg  RotationMatrix=[1 0 0; 0 1 0; 0 0 1]  Quaternion=[1 0 0 0]  TranslationMethod=StandardAxis  TranslationCartesianOffset=[0 0 0]  TranslationCartesianOffsetUnits=m  TranslationStandardAxis=-Z  TranslationStandardOffset=height_plane/2  TranslationStandardOffsetUnits=m  TranslationROffset=0  TranslationROffsetUnits=m  TranslationThetaOffset=0  TranslationThetaOffsetUnits=deg  TranslationZOffset=0  TranslationZOffsetUnits=m
  Plane Offset1 : sm_lib/Frames and Transforms/Rigid Transform  RotationMethod=None  FollAlignAxisA=+X  BaseAlignAxisA=+Y  FollAlignAxisB=+Y  BaseAlignAxisB=+Z  RotationStandardAxis=+Z  RotationAngle=0.0  RotationAngleUnits=deg  RotationArbitraryAxis=[0 0 1]  RotationSequenceAxes=FollowerAxes  RotationSequence=XYX  RotationSequenceAngles=[0 0 0]  RotationSequenceAnglesUnits=deg  RotationMatrix=[1 0 0; 0 1 0; 0 0 1]  Quaternion=[1 0 0 0]  TranslationMethod=StandardAxis  TranslationCartesianOffset=[0 0 0]  TranslationCartesianOffsetUnits=m  TranslationStandardAxis=-Z  TranslationStandardOffset=height_plane/2  TranslationStandardOffsetUnits=m  TranslationROffset=0  TranslationROffsetUnits=m  TranslationThetaOffset=0  TranslationThetaOffsetUnits=deg  TranslationZOffset=0  TranslationZOffsetUnits=m
  RB_Subsystem : Subsystem
  RF_Subsystem : Subsystem
  Simulink-PS Converter{1..12} (12 alike) : nesl_utility/Simulink-PS Converter  PhysicalDomain=network_engine_domain  SubClassName=ps_input  LeftPortType=input  RightPortType=output  PseudoPeriodic=off  Frequencies=[]  NoiseDistribution=none  NoiseParameters=[]  Unit=rad  AffineConversion=off  FilteringAndDerivatives=filter  SimscapeFilterOrder=2  InputFilterTimeConstant=0.001  UdotUserProvided=0
  Solver Configuration : nesl_utility/Solver Configuration  PhysicalDomain=network_engine_domain  SubClassName=solver  LeftPortType=input  RightPortType=generic  Tones=[]  Harmonics=[]  SimulateNoise=off  Profile=off  UseLocalSampling=off  EnableSwitchedLinearOptims=on  FrequencyDomain=off  UseCCode=off  RelTol=0.001  AbsTol=1e-06  MinStep=1e-09  ToWorkspace=off  RevertToSquareIcSolve=off  NumHomotopyIterations=100  PhasorMode=off  PhasorModeNumHarmonics=1  ConsistencySolver=NEWTON_FTOL  IndexReductionMethod=DerivativeReplacement  DoDC=off  ResidualTolerance=1e-09  ConsistencyTolSource=GLOBAL  ConsistencyAbsTol=0.001  ConsistencyRelTol=0.001  ConsistencyTolFactor=0.001  UseLocalSolver=off  LocalSolverChoice=NE_BACKWARD_EULER_ADVANCER  ResolveIndetEquations=on  FunctionEvalNumThread=1  LocalSolverSampleTime=0.001  DoFixedCost=off  MaxNonlinIter=3  MaxModeIter=2  ComputeImpulses=off  ImpulseIterations=2  LinearAlgebra=Sparse  LinearAlgebraNumThread=0  EquationFormulation=NE_TIME_EF  DelaysMemoryBudget=1024  AutomaticFiltering=on  FilteringTimeConstant=0.001  PartitionStorageMethod=AS_NEEDED  PartitionMemoryBudget=1024  PartitionMethod=FAST  MultibodyUseLocalSolver=off  MultibodyLocalSolverChoice=ODE1  MultibodyLocalSolverSampleTime=0.001
  Spatial Contact Force{,1..3} (4 alike) : sm_lib/Forces and Torques/Spatial Contact Force  NormalForceType=SmoothSpringDamper  NormalStiffness=contact_stiffness  NormalStiffnessUnits=N/m  NormalDamping=contact_damping  NormalDampingUnits=N/(m/s)  NormalTransitionRegionWidth=1e-4  NormalTransitionRegionWidthUnits=m  FrictionType=SmoothStickSlip  CoefficientOfStaticFriction=mu_s  CoefficientOfDynamicFriction=mu_k  FrictionalCriticalVelocity=mu_vth  FrictionalCriticalVelocityUnits=m/s  SenseContactSignal=off  SensePenetrationDepth=off  SenseSeparationDistance=off  SenseNormalForceMagnitude=on  SenseFrictionalForceMagnitude=on  SenseNormalVelocity=off  SenseTangentialVelocity=off  SenseContactBaseRotation=off  SenseContactBaseTranslation=off  SenseContactFollowerRotation=off  SenseContactFollowerTranslation=off  ZeroCrossDetectContactStartAndEnd=off
  Spherical Solid{,1..3} (4 alike) : sm_lib/Body Elements/Spherical Solid  SphereRadius=foot_z/2  SphereRadiusUnits=cm  ExportEntireGeometry=on  InertiaType=CalculateFromGeometry  BasedOnType=Mass  Density=1000  DensityUnits=kg/m^3  Mass=1  MassUnits=g  CenterOfMass=[0 0 0]  CenterOfMassUnits=m  MomentsOfInertia=[1 1 1]  MomentsOfInertiaUnits=kg*m^2  ProductsOfInertia=[0 0 0]  ProductsOfInertiaUnits=kg*m^2  GraphicType=FromGeometry  MarkerShape=Sphere  MarkerSize=10  GraphicVisPropType=SimpleVisualProperties  GraphicDiffuseColor=[0.5 0.5 0.5]  GraphicOpacity=1.0  GraphicSpecularColor=[0.5 0.5 0.5 1.0]  GraphicAmbientColor=[0.15 0.15 0.15 1.0]  GraphicEmissiveColor=[0.0 0.0 0.0 1.0]  GraphicShininess=75  DoExposeReferenceFrame=on  SerializedFrames=<Frames/>
  Terminator1 : Terminator
  Terminator10 : Terminator
  World Frame : sm_lib/Frames and Transforms/World Frame
  World Plane : sm_lib/Body Elements/Brick Solid  BrickDimensions="[plane_x plane_y  height_plane]"  BrickDimensionsUnits=m  ExportEntireGeometry=on  InertiaType=CalculateFromGeometry  BasedOnType=Density  Density=density  DensityUnits=kg/(m^3)  Mass=1  MassUnits=kg  CenterOfMass=[0 0 0]  CenterOfMassUnits=m  MomentsOfInertia=[1 1 1]  MomentsOfInertiaUnits=kg*m^2  ProductsOfInertia=[0 0 0]  ProductsOfInertiaUnits=kg*m^2  GraphicType=FromGeometry  MarkerShape=Sphere  MarkerSize=10  GraphicVisPropType=SimpleVisualProperties  GraphicDiffuseColor=[1.0 1.0 0.8]  GraphicOpacity=0.5  GraphicSpecularColor=[0.5 0.5 0.5 1.0]  GraphicAmbientColor=[0.15 0.15 0.15 1.0]  GraphicEmissiveColor=[0.0 0.0 0.0 1.0]  GraphicShininess=75  DoExposeReferenceFrame=on  SerializedFrames=<Frames/>
  wires:
  Bus Selector1/4 -> Simulink-PS Converter8/1  "<rf_alfa>"
  Bus Selector1/10 -> Simulink-PS Converter3/1  "<lf_alfa>"
  Bus Selector1/7 -> Simulink-PS Converter5/1  "<lb_alfa>"
  Bus Selector1/11 -> Simulink-PS Converter2/1  "<lf_beta>"
  Bus Selector1/9 -> Simulink-PS Converter6/1  "<lb_gamma>"
  Bus Selector1/6 -> Simulink-PS Converter9/1  "<rf_gamma>"
  Bus Selector1/3 -> Simulink-PS Converter12/1  "<rb_gamma>"
  leg_angle_watch/1 -> Bus Selector1/1
  Bus Selector1/5 -> Simulink-PS Converter7/1  "<rf_beta>"
  Bus Selector1/1 -> Simulink-PS Converter11/1  "<rb_alfa>"
  Bus Selector1/8 -> Simulink-PS Converter1/1  "<lb_beta>"
  Bus Selector1/12 -> Simulink-PS Converter4/1  "<lf_gamma>"
  Bus Selector1/2 -> Simulink-PS Converter10/1  "<rb_beta>"
  PS-Simulink Converter1/1 -> Add1/1
  PS-Simulink Converter7/1 -> Add1/4
  PS-Simulink Converter6/1 -> Add/4
  PS-Simulink Converter/1 -> Add/1
  PS-Simulink Converter4/1 -> Add/3
  PS-Simulink Converter2/1 -> Add/2
  Add1/1 -> Terminator1/1
  PS-Simulink Converter5/1 -> Add1/3
  Add/1 -> Terminator10/1
  PS-Simulink Converter3/1 -> Add1/2
  connections:
  Simulink-PS Converter6/RConn1 -- LB_Subsystem/LConn2
  Body_Subsystem/RConn4 -- LF_Subsystem/LConn1
  Spherical Solid2/RConn1 -- RF_Subsystem/RConn1
  Simulink-PS Converter7/RConn1 -- RF_Subsystem/LConn4
  Spherical Solid3/RConn1 -- RB_Subsystem/RConn1
  Body_Subsystem/RConn3 -- LB_Subsystem/LConn1
  Simulink-PS Converter10/RConn1 -- RB_Subsystem/LConn4
  Simulink-PS Converter5/RConn1 -- LB_Subsystem/LConn3
  Simulink-PS Converter11/RConn1 -- RB_Subsystem/LConn3
  Spherical Solid/RConn1 -- LF_Subsystem/RConn1
  LF_Subsystem/LConn4 -- Simulink-PS Converter2/RConn1
  Simulink-PS Converter12/RConn1 -- RB_Subsystem/LConn2
  RF_Subsystem/LConn1 -- Body_Subsystem/RConn2
  Solver Configuration/RConn1 -- Plane Offset1/LConn1 -- Mechanism Configuration/RConn1 -- Plane Offset/LConn1 -- World Frame/RConn1
  LF_Subsystem/LConn2 -- Simulink-PS Converter4/RConn1
  Simulink-PS Converter3/RConn1 -- LF_Subsystem/LConn3
  Simulink-PS Converter9/RConn1 -- RF_Subsystem/LConn2
  Simulink-PS Converter1/RConn1 -- LB_Subsystem/LConn4
  Plane Offset1/RConn1 -- Body_Subsystem/LConn1
  Body_Subsystem/RConn1 -- RB_Subsystem/LConn1
  Spherical Solid1/RConn1 -- LB_Subsystem/RConn1
  Simulink-PS Converter8/RConn1 -- RF_Subsystem/LConn3
  Spatial Contact Force1/LConn1 -- Spatial Contact Force/LConn1 -- World Plane/LConn1 -- Spatial Contact Force3/LConn1 -- Spatial Contact Force2/LConn1
  PS-Simulink Converter/LConn1 -- Spatial Contact Force/RConn2
  Spatial Contact Force1/RConn1 -- Spherical Solid1/LConn1
  PS-Simulink Converter4/LConn1 -- Spatial Contact Force2/RConn2
  PS-Simulink Converter1/LConn1 -- Spatial Contact Force/RConn3
  PS-Simulink Converter7/LConn1 -- Spatial Contact Force3/RConn3
  Spatial Contact Force3/RConn1 -- Spherical Solid3/LConn1
  Spatial Contact Force/RConn1 -- Spherical Solid/LConn1
  PS-Simulink Converter6/LConn1 -- Spatial Contact Force3/RConn2
  PS-Simulink Converter5/LConn1 -- Spatial Contact Force2/RConn3
  PS-Simulink Converter3/LConn1 -- Spatial Contact Force1/RConn3
  PS-Simulink Converter2/LConn1 -- Spatial Contact Force1/RConn2
  Spatial Contact Force2/RConn1 -- Spherical Solid2/LConn1
  World Plane/RConn1 -- Plane Offset/RConn1

== system leg_contral_from_joy/uart_send ==
  leg_angle : Inport
  Serial Configuration : instrumentseriallib/Serial Configuration  Priority=-200000  PortSel=/dev/ttyACM0  Port=/dev/ttyACM0  ComPort=/dev/ttyACM0  BaudRate=921600  DataBits=8  Parity=none  StopBits=1  ByteOrder=little-endian  FlowControl=none  Timeout=10  SimulateUsing=Interpreted execution  BlockInModel=on  aMode=1
      settings: LibrarySourceBlock=embeddedtargetslib/Host Communication/Serial Configuration
  Subsystem : Subsystem
  wires:
  leg_angle/1 -> Subsystem/1(In1)

== system leg_contral_from_joy/Joy_2_Leg_Angle/joy_aexs_out ==
  <axes> : Inport
  128_demux : Subsystem
  joy aexs Bus Creator : BusCreator  Inputs=8
  joy_aexs : Outport
  wires:
  128_demux/8(l_button_y) -> joy aexs Bus Creator/8  "l_button_y"
  128_demux/3(LT) -> joy aexs Bus Creator/3  "LT"
  128_demux/2(ly) -> joy aexs Bus Creator/2  "ly"
  128_demux/6(RT) -> joy aexs Bus Creator/6  "RT"
  128_demux/7(l_button_x) -> joy aexs Bus Creator/7  "l_button_x"
  128_demux/5(ry) -> joy aexs Bus Creator/5  "ry"
  128_demux/1(lx) -> joy aexs Bus Creator/1  "lx"
  128_demux/4(rx) -> joy aexs Bus Creator/4  "rx"
  <axes>/1 -> 128_demux/1(<axes>)
  joy aexs Bus Creator/1 -> joy_aexs/1

== system leg_contral_from_joy/Joy_2_Leg_Angle/joy_button_out ==
  <axes> : Inport
  128_demux : Subsystem
  joy aexs Bus Creator : BusCreator  Inputs=8
  joy_buttons : Outport
  wires:
  joy aexs Bus Creator/1 -> joy_buttons/1
  <axes>/1 -> 128_demux/1(<axes>)
  128_demux/1(A) -> joy aexs Bus Creator/1  "A"
  128_demux/2(B) -> joy aexs Bus Creator/2  "B"
  128_demux/3(X) -> joy aexs Bus Creator/3  "X"
  128_demux/4(Y) -> joy aexs Bus Creator/4  "Y"
  128_demux/5(LB) -> joy aexs Bus Creator/5  "LB"
  128_demux/6(RB) -> joy aexs Bus Creator/6  "RB"
  128_demux/7(BACK) -> joy aexs Bus Creator/7  "BACK"
  128_demux/8(START) -> joy aexs Bus Creator/8  "START"

== system leg_contral_from_joy/get_foot_step_lut/joy_aexs_out ==
  <axes> : Inport
  128_demux : Subsystem
  joy aexs Bus Creator : BusCreator  Inputs=8
  joy_aexs : Outport
  wires:
  128_demux/8(l_button_y) -> joy aexs Bus Creator/8  "l_button_y"
  128_demux/3(LT) -> joy aexs Bus Creator/3  "LT"
  128_demux/2(ly) -> joy aexs Bus Creator/2  "ly"
  128_demux/6(RT) -> joy aexs Bus Creator/6  "RT"
  128_demux/7(l_button_x) -> joy aexs Bus Creator/7  "l_button_x"
  128_demux/5(ry) -> joy aexs Bus Creator/5  "ry"
  128_demux/1(lx) -> joy aexs Bus Creator/1  "lx"
  128_demux/4(rx) -> joy aexs Bus Creator/4  "rx"
  <axes>/1 -> 128_demux/1(<axes>)
  joy aexs Bus Creator/1 -> joy_aexs/1

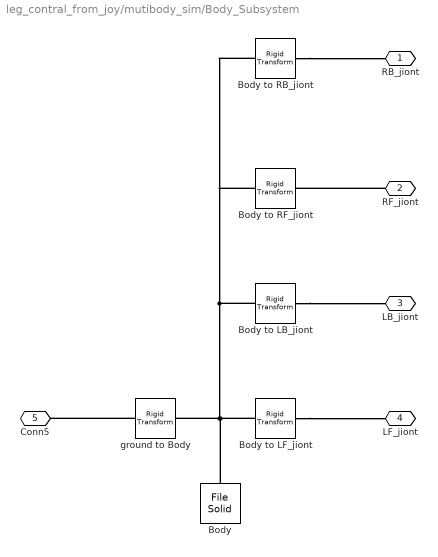
== system leg_contral_from_joy/mutibody_sim/Body_Subsystem ==
  Body : sm_lib/Body Elements/File Solid  ExtGeomFileName=STL/spotmicro_body_all_ly.STL  UnitType=Custom  ExtGeomFileUnits=mm  StepReaderType=HEX  ExportConvexHullGeometry=off  InertiaType=Custom  BasedOnType=Density  Density=1000  DensityUnits=kg/m^3  Mass=5500  MassUnits=g  CenterOfMass=[0 0 0]  CenterOfMassUnits=mm  MomentsOfInertia=[1 1 1]  MomentsOfInertiaUnits=kg*m^2  ProductsOfInertia=[0 0 0]  ProductsOfInertiaUnits=kg*m^2  GraphicType=FromGeometry  MarkerShape=Sphere  MarkerSize=10  GraphicVisPropType=SimpleVisualProperties  GraphicDiffuseColor=[0.5 0.5 0.5]  GraphicOpacity=1.0  GraphicSpecularColor=[0.5 0.5 0.5 1.0]  GraphicAmbientColor=[0.15 0.15 0.15 1.0]  GraphicEmissiveColor=[0.0 0.0 0.0 1.0]  GraphicShininess=75  DoExposeReferenceFrame=on  SerializedFrames=<Frames/>
  Body to LB_jiont : sm_lib/Frames and Transforms/Rigid Transform  RotationMethod=AlignedAxes  FollAlignAxisA=-Y  BaseAlignAxisA=+Z  FollAlignAxisB=+X  BaseAlignAxisB=-X  RotationStandardAxis=+X  RotationAngle=90  RotationAngleUnits=deg  RotationArbitraryAxis=[0 0 1]  RotationSequenceAxes=FollowerAxes  RotationSequence=XYX  RotationSequenceAngles=[0 0 0]  RotationSequenceAnglesUnits=deg  RotationMatrix=[1 0 0; 0 1 0; 0 0 1]  Quaternion=[1 0 0 0]  TranslationMethod=Cartesian  TranslationCartesianOffset=[39 70 6]  TranslationCartesianOffsetUnits=mm  TranslationStandardAxis=+Z  TranslationStandardOffset=100  TranslationStandardOffsetUnits=mm  TranslationROffset=0  TranslationROffsetUnits=m  TranslationThetaOffset=0  TranslationThetaOffsetUnits=deg  TranslationZOffset=0  TranslationZOffsetUnits=m
  Body to LF_jiont : sm_lib/Frames and Transforms/Rigid Transform  RotationMethod=StandardAxis  FollAlignAxisA=+Z  BaseAlignAxisA=+X  FollAlignAxisB=+Y  BaseAlignAxisB=+Z  RotationStandardAxis=+X  RotationAngle=-90  RotationAngleUnits=deg  RotationArbitraryAxis=[0 0 1]  RotationSequenceAxes=FollowerAxes  RotationSequence=XYX  RotationSequenceAngles=[0 0 0]  RotationSequenceAnglesUnits=deg  RotationMatrix=[1 0 0; 0 1 0; 0 0 1]  Quaternion=[1 0 0 0]  TranslationMethod=Cartesian  TranslationCartesianOffset=[39 -70 6]  TranslationCartesianOffsetUnits=mm  TranslationStandardAxis=+Z  TranslationStandardOffset=100  TranslationStandardOffsetUnits=mm  TranslationROffset=0  TranslationROffsetUnits=m  TranslationThetaOffset=0  TranslationThetaOffsetUnits=deg  TranslationZOffset=0  TranslationZOffsetUnits=m
  Body to RB_jiont : sm_lib/Frames and Transforms/Rigid Transform  RotationMethod=AlignedAxes  FollAlignAxisA=-Z  BaseAlignAxisA=+Y  FollAlignAxisB=+X  BaseAlignAxisB=-X  RotationStandardAxis=+X  RotationAngle=90  RotationAngleUnits=deg  RotationArbitraryAxis=[0 0 1]  RotationSequenceAxes=FollowerAxes  RotationSequence=XYX  RotationSequenceAngles=[0 0 0]  RotationSequenceAnglesUnits=deg  RotationMatrix=[1 0 0; 0 1 0; 0 0 1]  Quaternion=[1 0 0 0]  TranslationMethod=Cartesian  TranslationCartesianOffset=[-39 70 6]  TranslationCartesianOffsetUnits=mm  TranslationStandardAxis=+Z  TranslationStandardOffset=100  TranslationStandardOffsetUnits=mm  TranslationROffset=0  TranslationROffsetUnits=m  TranslationThetaOffset=0  TranslationThetaOffsetUnits=deg  TranslationZOffset=0  TranslationZOffsetUnits=m
  Body to RF_jiont : sm_lib/Frames and Transforms/Rigid Transform  RotationMethod=StandardAxis  FollAlignAxisA=+Z  BaseAlignAxisA=+X  FollAlignAxisB=+Y  BaseAlignAxisB=+Z  RotationStandardAxis=+X  RotationAngle=-90  RotationAngleUnits=deg  RotationArbitraryAxis=[0 0 1]  RotationSequenceAxes=FollowerAxes  RotationSequence=XYX  RotationSequenceAngles=[0 0 0]  RotationSequenceAnglesUnits=deg  RotationMatrix=[1 0 0; 0 1 0; 0 0 1]  Quaternion=[1 0 0 0]  TranslationMethod=Cartesian  TranslationCartesianOffset=[-39 -70 6]  TranslationCartesianOffsetUnits=mm  TranslationStandardAxis=+Z  TranslationStandardOffset=100  TranslationStandardOffsetUnits=mm  TranslationROffset=0  TranslationROffsetUnits=m  TranslationThetaOffset=0  TranslationThetaOffsetUnits=deg  TranslationZOffset=0  TranslationZOffsetUnits=m
  ground to Body : sm_lib/Frames and Transforms/Rigid Transform  RotationMethod=None  FollAlignAxisA=+X  BaseAlignAxisA=+Y  FollAlignAxisB=+Y  BaseAlignAxisB=+Z  RotationStandardAxis=+Z  RotationAngle=0.0  RotationAngleUnits=deg  RotationArbitraryAxis=[0 0 1]  RotationSequenceAxes=FollowerAxes  RotationSequence=XYX  RotationSequenceAngles=[0 0 0]  RotationSequenceAnglesUnits=deg  RotationMatrix=[1 0 0; 0 1 0; 0 0 1]  Quaternion=[1 0 0 0]  TranslationMethod=Cartesian  TranslationCartesianOffset=[0 0 250]  TranslationCartesianOffsetUnits=mm  TranslationStandardAxis=+Z  TranslationStandardOffset=0  TranslationStandardOffsetUnits=mm  TranslationROffset=0  TranslationROffsetUnits=m  TranslationThetaOffset=0  TranslationThetaOffsetUnits=deg  TranslationZOffset=0  TranslationZOffsetUnits=m
  RB_jiont : PMIOPort  Side=Right
  RF_jiont : PMIOPort  Port=2  Side=Right
  LB_jiont : PMIOPort  Port=3  Side=Right
  LF_jiont : PMIOPort  Port=4  Side=Right
  Conn5 : PMIOPort  Port=5  Side=Left
  connections:
  RF_jiont/RConn1 -- Body to RF_jiont/RConn1
  Body to LF_jiont/RConn1 -- LF_jiont/RConn1
  Body/RConn1 -- Body to LF_jiont/LConn1 -- ground to Body/RConn1 -- Body to RF_jiont/LConn1 -- Body to RB_jiont/LConn1 -- Body to LB_jiont/LConn1
  Body to LB_jiont/RConn1 -- LB_jiont/RConn1
  ground to Body/LConn1 -- Conn5/RConn1
  Body to RB_jiont/RConn1 -- RB_jiont/RConn1
